simulink subsystem "VCU_Subsystem"  (R2023b)
settings: Solver=VariableStepAuto  StartTime=0.0  StopTime=2  RelTol=1e-3
undefined symbols (not defined in the file or in its folder): canChannel
libraries: nesl_utility x9, fl_lib x8, ee_lib x6, canmsglib x3, canlib x2
settings Model: DefaultTestHarness=Charge_Contactor_Harness1  Creator=heyka  LastModifiedBy=mjmag
settings DebuggingCC: UnconnectedInputMsg=warning  UnconnectedOutputMsg=warning  UnconnectedLineMsg=warning
settings ModelReferenceCC: EnableRefExpFcnMdlSchedulingChecks=on
settings RTWCC: DLArmComputeVersion=19.05

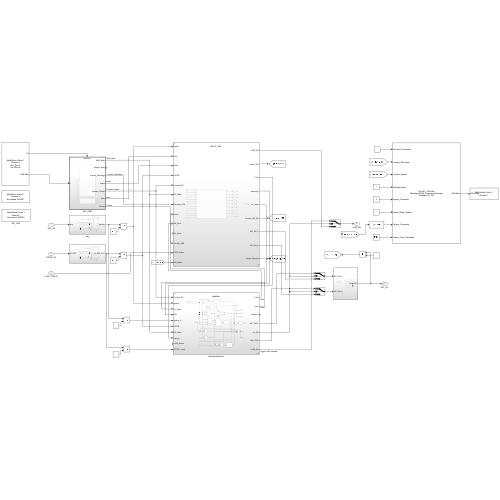
[thumbnail: Simulink's stored preview of the top-level diagram]
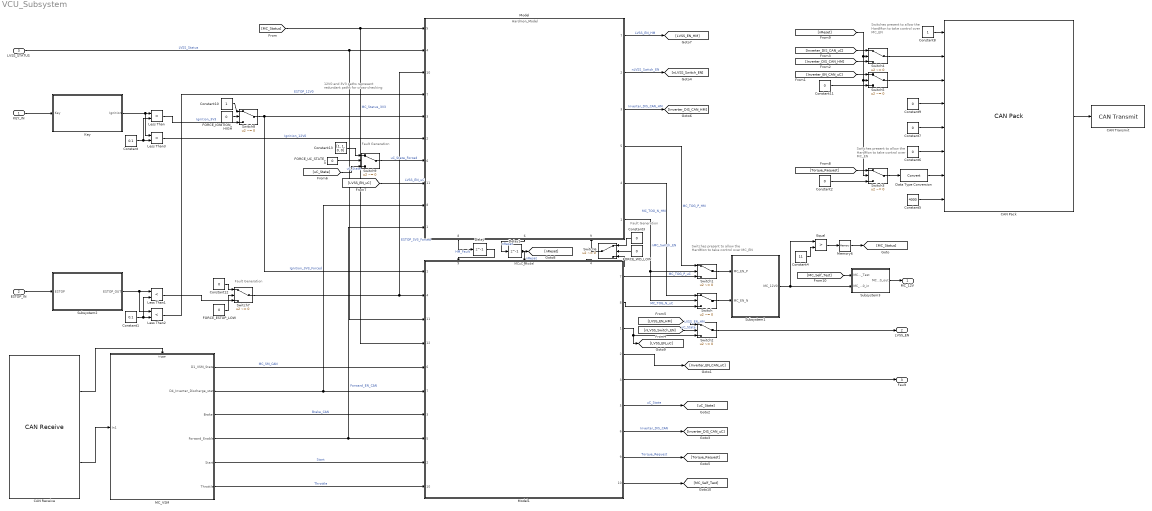
== system VCU_Subsystem ==
  note: Switches present to allow the HardMon to take control over MC_EN
  note: Switches present to allow the HardMon to take control over MC_EN
  note: Switches present to allow the HardMon to take control over MC_EN
  note: 12V0 and 3V3 paths represent redundant paths for cross-checking
  note: Fault Generation
  note: Fault Generation
  note: Fault Generation
  KEY_IN : Inport
  ESTOP_IN : Inport  Port=2
  LVSS_STATUS : Inport  Port=3  OutDataTypeStr=boolean
  CAN Pack : canmsglib/CAN Pack  CANdbFile=C:\Users\heyka\MATLAB\Projects\VCU_C\MC_CAN.dbc  MsgList=M192_Command_Message  MsgName=M192_Command_Message  MsgIDType=Standard (11-bit identifier)  MsgIdentifier=192  MsgLength=8  Remote=off  ApplyMinMax=off  BusOutput=off  SignalInfo={'Direction_Command','32','1','LE','unsigned','Standard','0','1','0','0','1';'Inverter_Discharge','41','1','LE','unsigned','Standard','0','1','0','0','1';'Inverter_Enable','40','1','LE','unsigned','Standard','0','1','0','0','1';'RollingCounter','44','4','LE','unsigned','Standard','0','1','0','0','15';'Speed_Command','16','16','LE','signed','Standard','0','1','0','-32768','32767';'Speed_Mode_Enable','42','1','LE','unsigned','Standard','0','1','0','0','1';'Torque_Command','0','16','LE','signed','Standard','0','0.1','0','-3276.8','3276.7';'Torque_Limit_Command','48','16','LE','signed','Standard','0','0.1','0','-3276.8','3276.7'}
      settings: LibrarySourceBlock=canlib/CAN Pack  DataFormat=CANdb specified signals
  CAN Receive : canlib/CAN Receive  BlockHandle=189.0004  Device=MathWorks Virtual 1 (Channel 2)  DeviceMenu=MathWorks Virtual 1 (Channel 2)  ObjConstructor=canChannel('MathWorks', 'Virtual 1', 2)  EnableStandardIDsFilter=off  StdIDsCombo=Allow all  StandardIDs=0  EnableExtendedIDsFilter=off  ExtIDsCombo=Allow all  ExtendedIDs=0  SampleTime=0.01  MsgsPerTimestep=all  InternalFilterUpdateStatus=on  BusOutput=off
  CAN Transmit : canlib/CAN Transmit  BlockHandle=596.0009  Device=MathWorks Virtual 1 (Channel 1)  DeviceMenu=MathWorks Virtual 1 (Channel 1)  ObjConstructor=canChannel('MathWorks', 'Virtual 1', 1)  EnableEventTransmit=off  EnablePeriodicTransmit=off  MessagePeriod=1.000
  Constant : Constant  Value=0.1
  Constant1 : Constant  Value=0.1
  Constant10 : Constant  OutDataTypeStr=boolean
  Constant{2..3,6..7,9,11} (6 alike) : Constant  Value=0
  Constant12 : Constant  Value=0  OutDataTypeStr=boolean
  Constant13 : Constant  Value=[1, 1, 0, 0]
  Constant4 : Constant  Value=11
  Constant5 : Constant  Value=4000
  Constant8 : Constant
  Data Type Conversion : DataTypeConversion  OutMin=[-32768]  OutMax=[32767]  SaturateOnIntegerOverflow=off  RndMeth=Floor
  Delay : Delay  DelayLength=1
  Delay1 : Delay  DelayLength=1
  Equal : RelationalOperator  Operator=>  OutDataTypeStr=boolean  RndMeth=Simplest  InputSameDT=off
  FORCE_ESTOP_LOW : Constant  Value=0
  FORCE_IGNITION_HIGH : Constant  Value=0
  FORCE_UC_STATE_3 : Constant  Value=0
  FORCE_WD_LOW : Constant  Value=0
  Key : Subsystem
  Less Than{,1..3} (4 alike) : RelationalOperator  Operator=<  OutDataTypeStr=boolean  RndMeth=Simplest  InputSameDT=off
  MC_VSM : Subsystem  TreatAsAtomicUnit=on
  Memory6 : Memory
  Model : ModelReference  ModelNameDialog=Hardmon_Model.slx  SimulationMode=Normal  ModelReferenceVersion=1.52
      settings: PortSchema="{\"entries\":[{\"content\":{\"sides\":[{\"content\":{\"connectorIds\":[\"In5\",\"In4\",\"In10\",\"In7\",\"In3\",\"In2\",\"In6\",\"In11\",\"In8\",\"In1\"]},\"type\":\"ConnectorPlacement.EquallySpacedRectSide\",\"uuid\":\"ce77178b-c7f8-493e-81d6-6e6e47cbf042\"},{\"content\":{\"connectorIds\":[\"Out7\",\"Out2\",\"Out3\",\"Out5\",\"Out4\",\"Out1\"],\"side\":\"RIGHT\"},\"type\":\"ConnectorPlacement.EquallySpacedRectSide\",\"uuid\":\"9ebffa51-7eff-4dd8-ac2f-4fbc962f2290\"},{\"content\":{\"side\":\"TOP\"},\"type\":\"ConnectorPlacement.EquallySpacedRectSide\",\"uuid\":\"a2dadd06-97c4-4e35-990a-e30edfa10790\"},{\"content\":{\"connectorIds\":[\"Out8\",\"Out6\",\"In9\"],\"side\":\"BOTTOM\"},\"type\":\"ConnectorPlacement.EquallySpacedRectSide\",\"uuid\":\"517832bd-7eeb-47f8-b142-e0ae288b30eb\"}]},\"type\":\"ConnectorPlacement.EquallySpacedConnector\",\"uuid\":\"ad9c7ae8-ba7b-4478-b44d-db7efe0b7c30\"}],\"packageUris\":[\"http://schema.mathworks.com/mf0/Connector/R2020b\"],\"version\":\"1.0\"}"
  Model1 : ModelReference  ModelNameDialog=MCuC_Model.slx  SimulationMode=Normal  ModelReferenceVersion=1.4
      settings: PortSchema="{\"entries\":[{\"content\":{\"sides\":[{\"content\":{\"connectorIds\":[\"In1\",\"In4\",\"In11\",\"In12\",\"In6\",\"In7\",\"In3\",\"In5\",\"In2\",\"In10\"]},\"type\":\"ConnectorPlacement.EquallySpacedRectSide\",\"uuid\":\"29930030-cffb-426b-9232-13bdddb5f01a\"},{\"content\":{\"connectorIds\":[\"Out7\",\"Out8\",\"Out1\",\"Out2\",\"Out3\",\"Out5\",\"Out6\",\"Out9\",\"Out10\"],\"side\":\"RIGHT\"},\"type\":\"ConnectorPlacement.EquallySpacedRectSide\",\"uuid\":\"e039672f-acfd-4e0d-841a-f9c7cf53404a\"},{\"content\":{\"connectorIds\":[\"In9\",\"In8\",\"Out4\"],\"side\":\"TOP\"},\"type\":\"ConnectorPlacement.EquallySpacedRectSide\",\"uuid\":\"ed3172ff-ca70-451f-85df-845f56faf5b0\"}]},\"type\":\"ConnectorPlacement.EquallySpacedConnector\",\"uuid\":\"b36a8819-9044-4231-aae1-023be34ba1c8\"}],\"packageUris\":[\"http://schema.mathworks.com/mf0/Connector/R2020b\"],\"version\":\"1.0\"}"
  Subsystem1 : Subsystem
  Subsystem2 : Subsystem
  Subsystem3 : Subsystem
  Switch{,1..5} (6 alike) : Switch  Criteria=u2 ~= 0  SaturateOnIntegerOverflow=off  InputSameDT=off
  Switch6 : Switch  Criteria=u2 ~= 0  OutDataTypeStr=Inherit: Inherit via back propagation  SaturateOnIntegerOverflow=off  InputSameDT=off
  Switch7 : Switch  Criteria=u2 ~= 0  OutDataTypeStr=boolean  SaturateOnIntegerOverflow=off  InputSameDT=off
  Switch8 : Switch  Criteria=u2 ~= 0  OutDataTypeStr=boolean  SaturateOnIntegerOverflow=off  InputSameDT=off
  Switch9 : Switch  Criteria=u2 ~= 0  OutDataTypeStr=Inherit: Inherit via back propagation  SaturateOnIntegerOverflow=off  InputSameDT=off
  MC_12V : Outport
  LVSS_EN : Outport  Port=2
  Fault : Outport  Port=3
  wires:
  Model/4 -> Switch/1  "MC_TOG_N_HM"
  Equal/1 -> Memory6/1
  ESTOP_IN/1 -> Subsystem2/1(ESTOP)
  MC_VSM/4(Forward_Enable) -> Model/1, Model1/5  "Forward_EN_CAN"
  Less Than2/1 -> Model/7  "ESTOP_12V0"
  Less Than3/1 -> Model/2  "Ignition_12V0"
  Switch/1 -> Subsystem1/2(MC_EN_N)
  Delay1/1 -> [nReset], Model1/8  "nReset"
  Switch1/1 -> Subsystem1/1(MC_EN_P)
  Constant1/1 -> Less Than1/2, Less Than2/2
  CAN Receive/2 -> MC_VSM/1(In1)
  Memory6/1 -> [MC_Status]
  Model1/7 -> Switch1/3  "MC_TOG_P_uC"
  Constant5/1 -> CAN Pack/8
  [Inverter_DIS_CAN_HM] -> Switch4/3
  Constant6/1 -> CAN Pack/6
  Key/1(Ignition) -> Less Than3/1, Less Than/1
  Switch5/1 -> CAN Pack/3
  Subsystem1/1(MC_12V0) -> Subsystem3/2(MC_12V0_in), Equal/1
  Constant8/1 -> CAN Pack/1
  Less Than1/1 -> Switch7/3
  Constant9/1 -> CAN Pack/4
  Constant7/1 -> CAN Pack/5
  MC_VSM/3(Brake) -> Model1/3  "Brake_CAN"
  Less Than/1 -> Switch8/3  "Ignition_3V3"
  Switch6/1 -> Model/9
  FORCE_WD_LOW/1 -> Switch6/2
  Data Type Conversion/1 -> CAN Pack/7
  Constant13/1 -> Switch9/1
  Model/8 -> Delay/1  "HM_Fault"
  FORCE_ESTOP_LOW/1 -> Switch7/2
  MC_VSM/6(Throttle) -> Model1/10  "Throttle"
  Subsystem3/1(MC_12V0_out) -> MC_12V/1
  Constant/1 -> Less Than/2, Less Than3/2
  MC_VSM/5(Start) -> Model1/2  "Start"
  FORCE_IGNITION_HIGH/1 -> Switch8/2
  Constant10/1 -> Switch8/1
  Model/1 -> Switch1/2, Switch/2  "nMC_Switch_EN"
  [LVSS_EN_uC] -> Model/11  "LVSS_EN_uC"
  MC_VSM/1(D1_VSM_State) -> Model1/6  "MC_SM_CAN"
  MC_VSM/2(D4_Inverter_Discharge_state) -> Model/8, Model1/7
  Model1/9 -> [Torque_Request]  "Torque_Request"
  Switch4/1 -> CAN Pack/2
  FORCE_UC_STATE_3/1 -> Switch9/2
  Model/3 -> [Inverter_DIS_CAN_HM]  "Inverter_DIS_CAN_HM"
  CAN Receive/1 -> MC_VSM/Trigger
  [MC_Status] -> Model/5, Model1/12  "MC_Status_3V3"
  Switch9/1 -> Model/6  "uC_State_Forced"
  [nReset] -> Switch3/2, Switch5/2, Switch4/2
  [Inverter_EN_CAN_uC] -> Switch5/1
  [nLVSS_Switch_EN] -> Switch2/2  "uC_State"
  Constant11/1 -> Switch5/3
  Constant2/1 -> Switch3/3
  Model1/3 -> Fault/1
  Constant4/1 -> Equal/2
  [Torque_Request] -> Switch3/1
  Constant3/1 -> Switch6/1
  Model1/8 -> Switch/3  "MC_TOG_N_uC"
  Subsystem2/1(ESTOP_OUT) -> Less Than1/1, Less Than2/1
  Switch7/1 -> Model/10, Model1/4  "ESTOP_3V3_Forced"
  [LVSS_EN_HM] -> Switch2/1  "LVSS_EN_HM"
  Constant12/1 -> Switch7/1
  [Inverter_DIS_CAN_uC] -> Switch4/1
  Model/5 -> Switch1/1  "MC_TOG_P_HM"
  Model/2 -> [nLVSS_Switch_EN]  "nLVSS_Switch_EN"
  Model1/6 -> [Inverter_DIS_CAN_uC]  "Inverter_DIS_CAN"
  Model1/1 -> [LVSS_EN_uC], Switch2/3
  Model1/4 -> Switch6/3
  LVSS_STATUS/1 -> Model/4, Model1/11  "LVSS_Status"
  Model/7 -> [LVSS_EN_HM]  "LVSS_EN_HM"
  Model1/2 -> [Inverter_EN_CAN_uC]
  Switch3/1 -> Data Type Conversion/1
  CAN Pack/1 -> CAN Transmit/1
  Model1/5 -> [uC_State]  "uC_State"
  [uC_State] -> Switch9/3  "uC_State"
  Model1/10 -> [MC_Self_Test]
  [MC_Self_Test] -> Subsystem3/1(MC_Self_Test)
  Switch8/1 -> Model/3, Model1/1  "Ignition_3V3_Forced"
  Switch2/1 -> LVSS_EN/1
  KEY_IN/1 -> Key/1(Key)
  Delay/1 -> Model1/9
  Model/6 -> Delay1/1  "nReset"

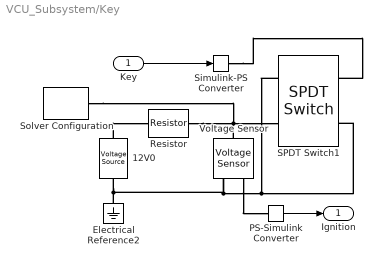
== system VCU_Subsystem/Key ==
  Key : Inport
  12V0 : ee_lib/Sources/Voltage Source  dc_voltage=12 V  ac_voltage=0 V  ac_shift=0 rad  ac_frequency=60 Hz  noise_mode=ee.enum.sources.noise.Disabled  PSD=0 V^2/Hz  sample_time=1e-3 s  repeatability=ee.enum.sources.repeatability.NotRepeatable  user_seed=0  auto_seed=3499211588  i_specify=off  i_priority=None  i=0 A  i_nominal_specify=off  i_nominal_unit=A  i_nominal_value=1  v_specify=off  v_priority=None  v=0 V  v_nominal_specify=off  v_nominal_unit=V  v_nominal_value=1
  Electrical Reference2 : fl_lib/Electrical/Electrical Elements/Electrical Reference
  PS-Simulink Converter : nesl_utility/PS-Simulink Converter  PhysicalDomain=network_engine_domain  SubClassName=ps_output  LeftPortType=input  RightPortType=output  PseudoPeriodic=off  Frequencies=[]  VectorFormat=inherit  Unit=inherit  AffineConversion=off
  Resistor : fl_lib/Electrical/Electrical Elements/Resistor  R=10000 Ohm  i_specify=off  i_priority=None  i=0 A  i_nominal_specify=off  i_nominal_unit=A  i_nominal_value=1  v_specify=off  v_priority=None  v=0 V  v_nominal_specify=off  v_nominal_unit=V  v_nominal_value=1
  SPDT Switch1 : ee_lib/Switches & Breakers/SPDT Switch  R_closed=0.01 Ohm  G_open=1e-10 S  Threshold=0.5 V  Width=0 V  model_dynamics=0  t_on=1e-3 s  t_off=1e-3 s  initial_vT=0 V
  Simulink-PS Converter : nesl_utility/Simulink-PS Converter  PhysicalDomain=network_engine_domain  SubClassName=ps_input  LeftPortType=input  RightPortType=output  PseudoPeriodic=off  Frequencies=[]  NoiseDistribution=none  NoiseParameters=[]  Unit=1  AffineConversion=off  FilteringAndDerivatives=provide  SimscapeFilterOrder=1  InputFilterTimeConstant=0.001  UdotUserProvided=0
  Solver Configuration : nesl_utility/Solver Configuration  PhysicalDomain=network_engine_domain  SubClassName=solver  LeftPortType=input  RightPortType=generic  Tones=[]  Harmonics=[]  SimulateNoise=off  Profile=off  UseLocalSampling=off  EnableSwitchedLinearOptims=on  FrequencyDomain=off  UseCCode=off  RelTol=0.001  AbsTol=0.001  MinStep=1e-09  ToWorkspace=off  RevertToSquareIcSolve=off  NumHomotopyIterations=100  PhasorMode=off  PhasorModeNumHarmonics=1  ConsistencySolver=NEWTON_XTOL_AFTER_FTOL  IndexReductionMethod=DerivativeReplacement  DoDC=off  ResidualTolerance=1e-09  ConsistencyTolSource=GLOBAL  ConsistencyAbsTol=0.001  ConsistencyRelTol=0.001  ConsistencyTolFactor=0.001  UseLocalSolver=off  LocalSolverChoice=NE_BACKWARD_EULER_ADVANCER  ResolveIndetEquations=on  FunctionEvalNumThread=1  LocalSolverSampleTime=0.001  DoFixedCost=off  MaxNonlinIter=3  MaxModeIter=2  ComputeImpulses=off  ImpulseIterations=2  LinearAlgebra=auto  LinearAlgebraNumThread=0  EquationFormulation=NE_TIME_EF  DelaysMemoryBudget=1024  AutomaticFiltering=on  FilteringTimeConstant=0.001  PartitionStorageMethod=AS_NEEDED  PartitionMemoryBudget=1024  PartitionMethod=ROBUST  MultibodyUseLocalSolver=off  MultibodyLocalSolverChoice=ODE1  MultibodyLocalSolverSampleTime=0.001
  Voltage Sensor : fl_lib/Electrical/Electrical Sensors/Voltage Sensor
  Ignition : Outport
  wires:
  PS-Simulink Converter/1 -> Ignition/1
  Key/1 -> Simulink-PS Converter/1
  connections:
  12V0/LConn1 -- Resistor/LConn1
  Resistor/RConn1 -- Solver Configuration/RConn1 -- Voltage Sensor/LConn1 -- SPDT Switch1/RConn2
  Electrical Reference2/LConn1 -- SPDT Switch1/RConn1 -- SPDT Switch1/LConn2 -- Voltage Sensor/RConn2 -- 12V0/RConn1
  Simulink-PS Converter/RConn1 -- SPDT Switch1/LConn1
  Voltage Sensor/RConn1 -- PS-Simulink Converter/LConn1

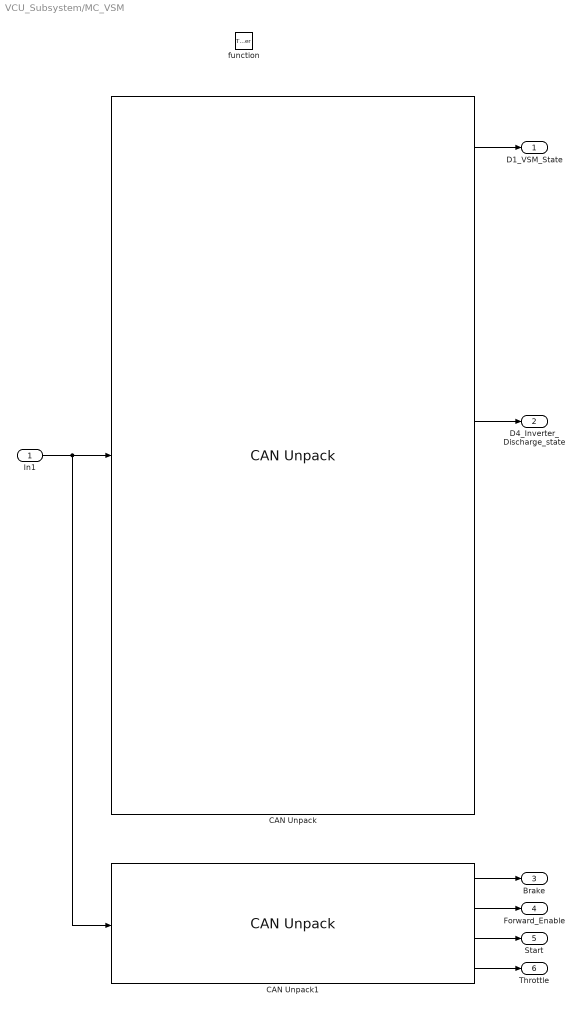
== system VCU_Subsystem/MC_VSM ==
  In1 : Inport
  function : TriggerPort  TriggerType=function-call  VariantControl=(inherit)
  CAN Unpack : canmsglib/CAN Unpack  CANdbFile=C:\Users\heyka\MATLAB\Projects\VCU_C\MC_CAN.dbc  MsgList=M170_Internal_States  MsgName=M170_Internal_States  MsgIDType=Standard (11-bit identifier)  MsgIdentifier=170  MsgLength=8  SignalInfo={'D1_PWM_Frequency','8','8','LE','unsigned','Standard','0','1','0','0','255';'D1_VSM_State','0','8','LE','unsigned','Standard','0','1','0','0','15';'D2_Inverter_State','16','8','LE','unsigned','Standard','0','1','0','0','255';'D3_Relay_1_Status','24','1','LE','unsigned','Standard','0','1','0','0','1';'D3_Relay_2_Status','25','1','LE','unsigned','Standard','0','1','0','0','1';'D3_Relay_3_Status','26','1','LE','unsigned','Standard','0','1','0','0','1';'D3_Relay_4_Status','27','1','LE','unsigned','Standard','0','1','0','0','1';'D3_Relay_5_Status','28','1','LE','unsigned','Standard','0','1','0','0','1';'D3_Relay_6_Status','29','1','LE','unsigned','Standard','0','1','0','0','1';'D4_Inverter_Discharge_State','37','3','LE','unsigned','Standard','0','1','0','0','7';'D4_Inverter_Run_Mode','32','1','LE','unsigned','Standard','0','1','0','0','1';'D5_Inverter_Command_Mode','40','1','LE','unsigned','Standard','0','1','0','0','1';'D5_Rolling_Counter','44','4','LE','unsigned','Standard','0','1','0','0','15';'D6_Inverter_Enable_Lockout','55','1','LE','unsigned','Standard','0','1','0','0','1';'D6_Inverter_Enable_State','48','1','LE','unsigned','Standard','0','1','0','0','1';'D6_Start_Mode_Active','54','1','LE','unsigned','Standard','0','1','0','0','1';'D7_BMS_Active','57','1','LE','unsigned','Standard','0','1','0','0','1';'D7_BMS_Torque_Limiting','58','1','LE','unsigned','Standard','0','1','0','0','1';'D7_Direction_Command','56','1','LE','unsigned','Standard','0','1','0','0','1';'D7_Low_Speed_Limiting','61','1','LE','unsigned','Standard','0','1','0','0','1';'D7_Max_Speed_Limiting','59','1','LE','unsigned','Standard','0','1','0','0','1'}  IDPort=off  TimestampPort=off  ErrorPort=off  RemotePort=off  LengthPort=off  StatusPort=off  ApplyMinMax=off
      settings: LibrarySourceBlock=canlib/CAN Unpack  DataFormat=CANdb specified signals
  CAN Unpack1 : canmsglib/CAN Unpack  CANdbFile=C:\Users\heyka\MATLAB\Projects\VCU_C\PRJDB.dbc  MsgList=N8_TPDO0  MsgName=N8_TPDO0  MsgIDType=Standard (11-bit identifier)  MsgIdentifier=392  MsgLength=5  SignalInfo={'Brake','1','16','LE','signed','Standard','0','1','0','0','494967295';'Forward_Enable','0','1','LE','unsigned','Standard','0','1','0','0','494967295';'Start','17','1','LE','unsigned','Standard','0','1','0','-Inf','Inf';'Throttle','18','16','LE','signed','Standard','0','1','0','-32768','32767'}  IDPort=off  TimestampPort=off  ErrorPort=off  RemotePort=off  LengthPort=off  StatusPort=off  ApplyMinMax=off
      settings: LibrarySourceBlock=canlib/CAN Unpack  DataFormat=CANdb specified signals
  D1_VSM_State : Outport
  D4_Inverter_Discharge_state : Outport  Port=2
  Brake : Outport  Port=3  OutDataTypeStr=int16
  Forward_Enable : Outport  Port=4  OutDataTypeStr=boolean
  Start : Outport  Port=5  OutDataTypeStr=boolean
  Throttle : Outport  Port=6  OutDataTypeStr=int16
  wires:
  In1/1 -> CAN Unpack1/1, CAN Unpack/1
  CAN Unpack/2 -> D1_VSM_State/1
  CAN Unpack/10 -> D4_Inverter_Discharge_state/1
  CAN Unpack1/1 -> Brake/1
  CAN Unpack1/2 -> Forward_Enable/1
  CAN Unpack1/3 -> Start/1
  CAN Unpack1/4 -> Throttle/1

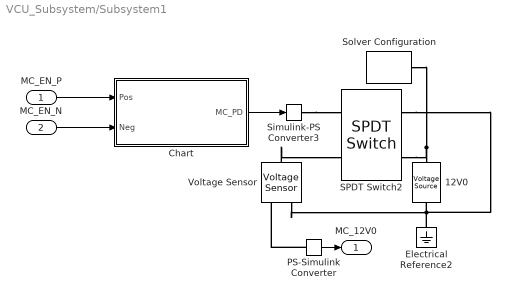
== system VCU_Subsystem/Subsystem1 ==
  MC_EN_P : Inport
  MC_EN_N : Inport  Port=2
  12V0 : ee_lib/Sources/Voltage Source  dc_voltage=12 V  ac_voltage=0 V  ac_shift=0 rad  ac_frequency=60 Hz  noise_mode=ee.enum.sources.noise.Disabled  PSD=0 V^2/Hz  sample_time=1e-3 s  repeatability=ee.enum.sources.repeatability.NotRepeatable  user_seed=0  auto_seed=3890346746  i_specify=off  i_priority=None  i=0 A  i_nominal_specify=off  i_nominal_unit=A  i_nominal_value=1  v_specify=off  v_priority=None  v=0 V  v_nominal_specify=off  v_nominal_unit=V  v_nominal_value=1
  Chart : Stateflow chart  TreatAsAtomicUnit=on
  Electrical Reference2 : fl_lib/Electrical/Electrical Elements/Electrical Reference
  PS-Simulink Converter : nesl_utility/PS-Simulink Converter  PhysicalDomain=network_engine_domain  SubClassName=ps_output  LeftPortType=input  RightPortType=output  PseudoPeriodic=off  Frequencies=[]  VectorFormat=inherit  Unit=inherit  AffineConversion=off
  SPDT Switch2 : ee_lib/Switches & Breakers/SPDT Switch  R_closed=0.01 Ohm  G_open=1e-6 S  Threshold=0.5 V  Width=0 V  model_dynamics=0  t_on=1e-3 s  t_off=1e-3 s  initial_vT=0 V
  Simulink-PS Converter3 : nesl_utility/Simulink-PS Converter  PhysicalDomain=network_engine_domain  SubClassName=ps_input  LeftPortType=input  RightPortType=output  PseudoPeriodic=off  Frequencies=[]  NoiseDistribution=none  NoiseParameters=[]  Unit=1  AffineConversion=off  FilteringAndDerivatives=provide  SimscapeFilterOrder=1  InputFilterTimeConstant=0.001  UdotUserProvided=0
  Solver Configuration : nesl_utility/Solver Configuration  PhysicalDomain=network_engine_domain  SubClassName=solver  LeftPortType=input  RightPortType=generic  Tones=[]  Harmonics=[]  SimulateNoise=off  Profile=off  UseLocalSampling=off  EnableSwitchedLinearOptims=on  FrequencyDomain=off  UseCCode=off  RelTol=0.001  AbsTol=0.001  MinStep=1e-09  ToWorkspace=off  RevertToSquareIcSolve=off  NumHomotopyIterations=100  PhasorMode=off  PhasorModeNumHarmonics=1  ConsistencySolver=NEWTON_XTOL_AFTER_FTOL  IndexReductionMethod=DerivativeReplacement  DoDC=off  ResidualTolerance=1e-09  ConsistencyTolSource=GLOBAL  ConsistencyAbsTol=0.001  ConsistencyRelTol=0.001  ConsistencyTolFactor=0.001  UseLocalSolver=off  LocalSolverChoice=NE_BACKWARD_EULER_ADVANCER  ResolveIndetEquations=on  FunctionEvalNumThread=1  LocalSolverSampleTime=0.001  DoFixedCost=off  MaxNonlinIter=3  MaxModeIter=2  ComputeImpulses=off  ImpulseIterations=2  LinearAlgebra=auto  LinearAlgebraNumThread=0  EquationFormulation=NE_TIME_EF  DelaysMemoryBudget=1024  AutomaticFiltering=on  FilteringTimeConstant=0.001  PartitionStorageMethod=AS_NEEDED  PartitionMemoryBudget=1024  PartitionMethod=ROBUST  MultibodyUseLocalSolver=off  MultibodyLocalSolverChoice=ODE1  MultibodyLocalSolverSampleTime=0.001
  Voltage Sensor : fl_lib/Electrical/Electrical Sensors/Voltage Sensor
  MC_12V0 : Outport
  wires:
  MC_EN_P/1 -> Chart/1(Pos)
  MC_EN_N/1 -> Chart/2(Neg)
  Chart/1(MC_PD) -> Simulink-PS Converter3/1
  PS-Simulink Converter/1 -> MC_12V0/1
  connections:
  Simulink-PS Converter3/RConn1 -- SPDT Switch2/LConn1
  PS-Simulink Converter/LConn1 -- Voltage Sensor/RConn1
  Electrical Reference2/LConn1 -- 12V0/RConn1 -- Voltage Sensor/RConn2 -- SPDT Switch2/RConn1
  SPDT Switch2/RConn2 -- Solver Configuration/RConn1 -- 12V0/LConn1
  Voltage Sensor/LConn1 -- SPDT Switch2/LConn2

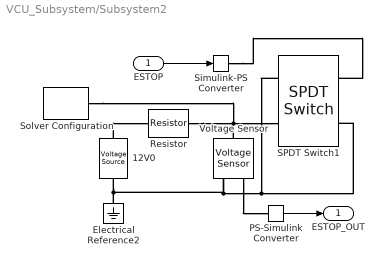
== system VCU_Subsystem/Subsystem2 ==
  ESTOP : Inport
  12V0 : ee_lib/Sources/Voltage Source  dc_voltage=12 V  ac_voltage=0 V  ac_shift=0 rad  ac_frequency=60 Hz  noise_mode=ee.enum.sources.noise.Disabled  PSD=0 V^2/Hz  sample_time=1e-3 s  repeatability=ee.enum.sources.repeatability.NotRepeatable  user_seed=0  auto_seed=545404223  i_specify=off  i_priority=None  i=0 A  i_nominal_specify=off  i_nominal_unit=A  i_nominal_value=1  v_specify=off  v_priority=None  v=0 V  v_nominal_specify=off  v_nominal_unit=V  v_nominal_value=1
  Electrical Reference2 : fl_lib/Electrical/Electrical Elements/Electrical Reference
  PS-Simulink Converter : nesl_utility/PS-Simulink Converter  PhysicalDomain=network_engine_domain  SubClassName=ps_output  LeftPortType=input  RightPortType=output  PseudoPeriodic=off  Frequencies=[]  VectorFormat=inherit  Unit=inherit  AffineConversion=off
  Resistor : fl_lib/Electrical/Electrical Elements/Resistor  R=10000 Ohm  i_specify=off  i_priority=None  i=0 A  i_nominal_specify=off  i_nominal_unit=A  i_nominal_value=1  v_specify=off  v_priority=None  v=0 V  v_nominal_specify=off  v_nominal_unit=V  v_nominal_value=1
  SPDT Switch1 : ee_lib/Switches & Breakers/SPDT Switch  R_closed=0.01 Ohm  G_open=1e-10 S  Threshold=0.5 V  Width=0 V  model_dynamics=0  t_on=1e-3 s  t_off=1e-3 s  initial_vT=0 V
  Simulink-PS Converter : nesl_utility/Simulink-PS Converter  PhysicalDomain=network_engine_domain  SubClassName=ps_input  LeftPortType=input  RightPortType=output  PseudoPeriodic=off  Frequencies=[]  NoiseDistribution=none  NoiseParameters=[]  Unit=1  AffineConversion=off  FilteringAndDerivatives=provide  SimscapeFilterOrder=1  InputFilterTimeConstant=0.001  UdotUserProvided=0
  Solver Configuration : nesl_utility/Solver Configuration  PhysicalDomain=network_engine_domain  SubClassName=solver  LeftPortType=input  RightPortType=generic  Tones=[]  Harmonics=[]  SimulateNoise=off  Profile=off  UseLocalSampling=off  EnableSwitchedLinearOptims=on  FrequencyDomain=off  UseCCode=off  RelTol=0.001  AbsTol=0.001  MinStep=1e-09  ToWorkspace=off  RevertToSquareIcSolve=off  NumHomotopyIterations=100  PhasorMode=off  PhasorModeNumHarmonics=1  ConsistencySolver=NEWTON_XTOL_AFTER_FTOL  IndexReductionMethod=DerivativeReplacement  DoDC=off  ResidualTolerance=1e-09  ConsistencyTolSource=GLOBAL  ConsistencyAbsTol=0.001  ConsistencyRelTol=0.001  ConsistencyTolFactor=0.001  UseLocalSolver=off  LocalSolverChoice=NE_BACKWARD_EULER_ADVANCER  ResolveIndetEquations=on  FunctionEvalNumThread=1  LocalSolverSampleTime=0.001  DoFixedCost=off  MaxNonlinIter=3  MaxModeIter=2  ComputeImpulses=off  ImpulseIterations=2  LinearAlgebra=auto  LinearAlgebraNumThread=0  EquationFormulation=NE_TIME_EF  DelaysMemoryBudget=1024  AutomaticFiltering=on  FilteringTimeConstant=0.001  PartitionStorageMethod=AS_NEEDED  PartitionMemoryBudget=1024  PartitionMethod=ROBUST  MultibodyUseLocalSolver=off  MultibodyLocalSolverChoice=ODE1  MultibodyLocalSolverSampleTime=0.001
  Voltage Sensor : fl_lib/Electrical/Electrical Sensors/Voltage Sensor
  ESTOP_OUT : Outport
  wires:
  PS-Simulink Converter/1 -> ESTOP_OUT/1
  ESTOP/1 -> Simulink-PS Converter/1
  connections:
  12V0/LConn1 -- Resistor/LConn1
  Voltage Sensor/LConn1 -- SPDT Switch1/RConn2 -- Resistor/RConn1 -- Solver Configuration/RConn1
  SPDT Switch1/LConn2 -- 12V0/RConn1 -- Electrical Reference2/LConn1 -- Voltage Sensor/RConn2 -- SPDT Switch1/RConn1
  Simulink-PS Converter/RConn1 -- SPDT Switch1/LConn1
  Voltage Sensor/RConn1 -- PS-Simulink Converter/LConn1

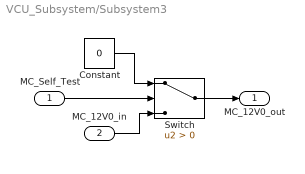
== system VCU_Subsystem/Subsystem3 ==
  MC_Self_Test : Inport
  MC_12V0_in : Inport  Port=2
  Constant : Constant  Value=0
  Switch : Switch  Criteria=u2 > Threshold  SaturateOnIntegerOverflow=off  InputSameDT=off
  MC_12V0_out : Outport
  wires:
  MC_12V0_in/1 -> Switch/3
  Constant/1 -> Switch/1
  Switch/1 -> MC_12V0_out/1
  MC_Self_Test/1 -> Switch/2

== stateflow chart VCU_Subsystem/Subsystem1/Chart ==
  state Relay_Open
    MC_PD = 0;
  state Relay_Close
    MC_PD = 1;
  (default) -> Relay_Open
  Relay_Open -> Relay_Close : [Pos == 1 && Neg == 0]
  Relay_Close -> Relay_Open : [Pos == 0 && Neg == 1]
  data: Pos input; MC_PD output =0; Neg input
